simulink model "flightControlSystem"  (R2024a)
settings: Solver=ode3  StartTime=0  StopTime=TFinal  FixedStep=Ts  RelTol=1e-3  EnableMultiTasking=on
undefined symbols (not defined in the file): codertarget, Controller, DiscIntNeverNeededParam, Discrete, Estimator, g, gray, init, Sensors, Time, Ts, var_acc_angle_N, var_bias_gyr_N, var_gyro_p_N, Vehicle
libraries: simulink x37, visiontextngfix x12, slpidlib x4, ctrlSharedLib x4, sharedtransform x3, visionconversions x1, parrotlib x1
(part 3 of 3)

== matlab function flightControlSystem/Image Processing System1/MATLAB Function3 ==
  data: pathold input; N input; centroid input; centroid_blk input; area_l input; area_r input; roiangle output; angle input; roicord_l output size=[1 6]; roicord_r output size=[1 6]; blackcord_l output; blackcord_r output; speed output
function [roiangle, roicord_l, roicord_r,blackcord_l , blackcord_r, speed] = ReigonofInterest( pathold, N, centroid, centroid_blk, area_l, area_r, angle)
path=[centroid 80 60];
% [row,~]=size(path);
x=[80 60];
y=[path(1,1) path(1,2)];
d1=norm(x-y);
y=[path(1,3) path(1,4)];
d2=norm(x-y);
x=[path(1,1) path(1,2)];
y=[80 60];
pathdis=norm(x-y)
if pathdis<6 && pathdis >=4
    speed=0.25;
elseif pathdis<4
    path=[centroid_blk 80 60];
    speed=1.2;
elseif pathdis<20 && pathdis >=10
    speed=pathdis/300
else
    speed=pathdis/250
end

if (pathold(1,1)+pathold(1,2)+pathold(1,3)+pathold(1,4))~=0
pendis=abs((pathold(1,3) - pathold(1,1)) * (pathold(1,2) - 60) - (pathold(1,1) - 80) * (pathold(1,4) - pathold(1,2)))./sqrt((pathold(1,3) - pathold(1,1)) ^ 2 + (pathold(1,4) - pathold(1,2)) ^ 2)
x=[pathold(1,1) pathold(1,3)];
y=[pathold(1,2) pathold(1,4)];
pathdisold=norm(x-y);
anglecorr=pendis/pathdisold;
pendis_cen=abs((pathold(1,3) - pathold(1,1)) * (pathold(1,2) - centroid(2)) - (pathold(1,1) - centroid(1)) * (pathold(1,4) - pathold(1,2)))./sqrt((pathold(1,3) - pathold(1,1)) ^ 2 + (pathold(1,4) - pathold(1,2)) ^ 2)
    if (pendis<= 10 || (pendis>= 10 && pendis_cen>=5)) && pathdis ~=1
    
    
    if   (path(1,1)+path(1,2)+path(1,3)+path(1,4))~=0 && d1>=d2 
    
   
    
        pendis=abs((path(1,3) - path(1,1)) * (path(1,2) - 60) - (path(1,1) - 80) * (path(1,4) - path(1,2)))./sqrt((path(1,3) - path(1,1)) ^ 2 + (path(1,4) - path(1,2)) ^ 2);
        x=[path(1,1) path(1,3)];
        y=[path(1,2) path(1,4)];
        pathdis=norm(x-y);
        anglecorr=pendis/pathdis;
    
        a = [-80*(path(1,3)-path(1,1)) - 60*(path(1,4)-path(1,2)) ;  -path(1,2)*(path(1,3)-path(1,1)) + path(1,1)*(path(1,4)-path(1,2))]; 
        b = [path(1,3) - path(1,1), path(1,4) - path(1,2) ;  path(1,2) - path(1,4), path(1,3) - path(1,1)];
        projpoint = -(b\a)-[80,60];
    
        if projpoint(1)<0 && angle>-1.5708 && angle<1.5708
            anglecorr=-anglecorr;
        elseif  projpoint(1)>0 && (angle<-1.5708 || angle>1.5708)
            anglecorr=-anglecorr;
        elseif projpoint(1)==0 && projpoint(2)>0 && angle==1.5708 
            anglecorr=-anglecorr;
        elseif projpoint(1)==0 && projpoint(2)<0 && angle==-1.5708 
            anglecorr=-anglecorr;
        end
    
    
        v1 = [path(1,3) - path(1,1) , path( 1,4)- path(1,2)];
        v2 = [ 0, 1];
        roiangle = acos(dot(v1,v2)/(norm(v1)*norm(v2))) +anglecorr;
        
        if path(1,1)<80
            roiangle=-roiangle;
        end
    
        
    elseif  (path(1,1)+path(1,2)+path(1,3)+path(1,4))~=0 && d2>=d1 
    
        pendis=abs((path(1,3) - path(1,1)) * (path(1,2) - 60) - (path(1,1) - 80) * (path(1,4) - path(1,2)))./sqrt((path(1,3) - path(1,1)) ^ 2 + (path(1,4) - path(1,2)) ^ 2);
        x=[path(1,1) path(1,3)];
        y=[path(1,2) path(1,4)];
        pathdis=norm(x-y);
        anglecorr=pendis/pathdis;
    
        a = [-80*(path(1,3)-path(1,1)) - 60*(path(1,4)-path(1,2)) ;  -path(1,2)*(path(1,3)-path(1,1)) + path(1,1)*(path(1,4)-path(1,2))]; 
        b = [path(1,3) - path(1,1), path(1,4) - path(1,2) ;  path(1,2) - path(1,4), path(1,3) - path(1,1)];
        projpoint = -(b\a)-[80,60];
    
        if projpoint(1)<0 && angle>-1.5708 && angle<1.5708
            anglecorr=-anglecorr;
        elseif  projpoint(1)>0 && (angle<-1.5708 || angle>1.5708)
            anglecorr=-anglecorr;
        elseif projpoint(1)==0 && projpoint(2)>0 && angle==1.5708 
            anglecorr=-anglecorr;
        elseif projpoint(1)==0 && projpoint(2)<0 && angle==-1.5708 
            anglecorr=-anglecorr;
        end
    
        v1 = [path(1,1) - path(1,3) , path( 1,2)- path(1,4)];
        v2 = [ 0, 1];
        roiangle = acos(dot(v1,v2)/(norm(v1)*norm(v2))) +anglecorr;
    
        if path(1,1)<80
            roiangle=-roiangle;
        end
    
    
    
    elseif (path(1,1)+path(1,2)+path(1,3)+path(1,4))~=0
    
        pendis=abs((path(1,3) - path(1,1)) * (path(1,2) - 60) - (path(1,1) - 80) * (path(1,4) - path(1,2)))./sqrt((path(1,3) - path(1,1)) ^ 2 + (path(1,4) - path(1,2)) ^ 2);
        x=[path(1,1) path(1,3)];
        y=[path(1,2) path(1,4)];
        pathdis=norm(x-y);
        anglecorr=pendis/pathdis;
    
        a = [-80*(path(1,3)-path(1,1)) - 60*(path(1,4)-path(1,2)) ;  -path(1,2)*(path(1,3)-path(1,1)) + path(1,1)*(path(1,4)-path(1,2))]; 
        b = [path(1,3) - path(1,1), path(1,4) - path(1,2) ;  path(1,2) - path(1,4), path(1,3) - path(1,1)];
        projpoint = -(b\a)-[80,60];
    
        if projpoint(1)<0 && angle>-1.5708 && angle<1.5708
            anglecorr=-anglecorr;
        elseif  projpoint(1)>0 && (angle<-1.5708 || angle>1.5708)
            anglecorr=-anglecorr;
        elseif projpoint(1)==0 && projpoint(2)>0 && angle==1.5708 
            anglecorr=-anglecorr;
        elseif projpoint(1)==0 && projpoint(2)<0 && angle==-1.5708 
            anglecorr=-anglecorr;
        end
    
        v1 = [path(1,3) - path(1,1) , path( 1,4)- path(1,2)];
        v2 = [ 0, path(1,1) - path(1,2)];
        roiangle = acos(dot(v1,v2)/(norm(v1)*norm(v2))) +anglecorr;
    
    
    else
            roiangle=angle;
        speed=0.3;
    end
    else
        a = [-80*(pathold(1,3)-pathold(1,1)) - 60*(pathold(1,4)-pathold(1,2)) ;  -pathold(1,2)*(pathold(1,3)-pathold(1,1)) + pathold(1,1)*(pathold(1,4)-pathold(1,2))]; 
        b = [pathold(1,3) - pathold(1,1), pathold(1,4) - pathold(1,2) ;  pathold(1,2) - pathold(1,4), pathold(1,3) - pathold(1,1)];
        projpoint = -(b\a)-[80,60];
    
        if projpoint(1)<0 && angle>-1.5708 && angle<1.5708
            anglecorr=-anglecorr;
        elseif  projpoint(1)>0 && (angle<-1.5708 || angle>1.5708)
            anglecorr=-anglecorr;
        elseif projpoint(1)==0 && projpoint(2)>0 && angle==1.5708 
            anglecorr=-anglecorr;
        elseif projpoint(1)==0 && projpoint(2)<0 && angle==-1.5708 
            anglecorr=-anglecorr;
        end
    
        roiangle=angle+anglecorr/10;
        speed=0.2;
    end
else
    roiangle=angle;
    speed=0.1;
end
n=10;
m=25;
l=25;
xc=80;
yc=60;

x0=xc-l*sin(roiangle);
y0=yc+l*cos(roiangle);
x1=xc+m*sin(roiangle);
y1=yc-m*cos(roiangle);
xr=x1+n*(y0-y1)/m;
yr=y1+n*(x1-x0)/m;
xl=x1-n*(y0-y1)/m;
yl=y1-n*(x1-x0)/m;


roicord_l=[x0 y0 xl yl x1 y1] ;
roicord_r=[x0 y0 x1 y1 xr yr];


n=60;
m=100;
l=0;
xc=80;
yc=60;


x0=xc-l*sin(roiangle+pi);
y0=yc+l*cos(roiangle+pi);
x1=xc+m*sin(roiangle+pi);
y1=yc-m*cos(roiangle+pi);
xr=x1+n*(y0-y1)/m;
yr=y1+n*(x1-x0)/m;
xl=x1-n*(y0-y1)/m;
yl=y1-n*(x1-x0)/m;


blackcord_l=[x0 y0 xl yl x1 y1] ;
blackcord_r=[x0 y0 x1 y1 xr yr];
